simulink model "enable_test"  (Simulink 9.0)
settings: Solver=FixedStepDiscrete  StartTime=0.0  StopTime=1  FixedStep=1.000000  MaxStep=1  RelTol=1e-3  EnableMultiTasking=on
undefined symbols (not defined in the file): DiscIntNeverNeededParam
libraries: simulink x1
settings Model: SuppressorTable=22 serialization::archive 11 0 6 0 0 0 0 0  Creator=arnaud  LastModifiedBy=hbourbou
settings DataIOCC: ExternalInput=xin  LimitDataPoints=on  SaveFormat=StructureWithTime
settings DebuggingCC: UnderspecifiedInitializationDetection=Simplified  MergeDetectMultiDrivingBlocksExec=error  SolverPrmCheckMsg=warning
settings GRTTargetCC: GeneratePreprocessorConditionals=Disable all
settings ConfigComp: CovSFcnEnable=off

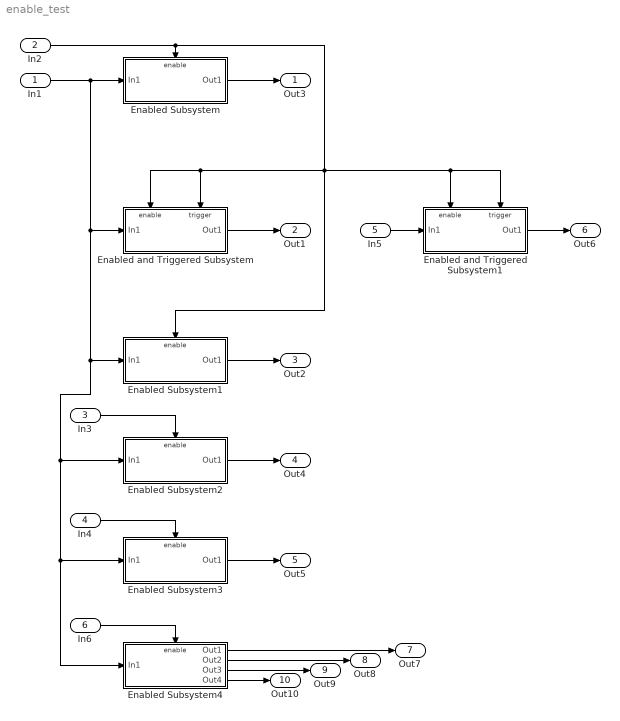
== system enable_test ==
  In1 : Inport
  In2 : Inport  Port=2  OutDataTypeStr=boolean
  In3 : Inport  Port=3  OutDataTypeStr=int8  PortDimensions=3
  In4 : Inport  Port=4  OutDataTypeStr=double
  In5 : Inport  Port=5
  In6 : Inport  Port=6  OutDataTypeStr=double
  Enabled Subsystem : Subsystem  TreatAsAtomicUnit=on
  Enabled Subsystem1 : Subsystem  TreatAsAtomicUnit=on
  Enabled Subsystem2 : Subsystem  TreatAsAtomicUnit=on
  Enabled Subsystem3 : Subsystem  TreatAsAtomicUnit=on
  Enabled Subsystem4 : Subsystem  TreatAsAtomicUnit=on
  Enabled and Triggered Subsystem : Subsystem  TreatAsAtomicUnit=on
  Enabled and Triggered Subsystem1 : Subsystem  TreatAsAtomicUnit=on
  Out3 : Outport
  Out1 : Outport  Port=2
  Out2 : Outport  Port=3
  Out4 : Outport  Port=4
  Out5 : Outport  Port=5
  Out6 : Outport  Port=6
  Out7 : Outport  Port=7
  Out8 : Outport  Port=8
  Out9 : Outport  Port=9
  Out10 : Outport  Port=10
  wires:
  Enabled Subsystem/1(Out1) -> Out3/1
  In2/1 -> Enabled and Triggered Subsystem1/Trigger, Enabled and Triggered Subsystem1/Enable, Enabled Subsystem1/Enable, Enabled and Triggered Subsystem/Trigger, Enabled and Triggered Subsystem/Enable, Enabled Subsystem/Enable
  Enabled and Triggered Subsystem/1(Out1) -> Out1/1
  Enabled Subsystem1/1(Out1) -> Out2/1
  Enabled Subsystem2/1(Out1) -> Out4/1
  Enabled Subsystem3/1(Out1) -> Out5/1
  In3/1 -> Enabled Subsystem2/Enable
  In4/1 -> Enabled Subsystem3/Enable
  Enabled and Triggered Subsystem1/1(Out1) -> Out6/1
  In5/1 -> Enabled and Triggered Subsystem1/1(In1)
  In1/1 -> Enabled Subsystem4/1(In1), Enabled Subsystem3/1(In1), Enabled Subsystem2/1(In1), Enabled Subsystem1/1(In1), Enabled and Triggered Subsystem/1(In1), Enabled Subsystem/1(In1)
  Enabled Subsystem4/1(Out1) -> Out7/1
  In6/1 -> Enabled Subsystem4/Enable
  Enabled Subsystem4/2(Out2) -> Out8/1
  Enabled Subsystem4/3(Out3) -> Out9/1
  Enabled Subsystem4/4(Out4) -> Out10/1

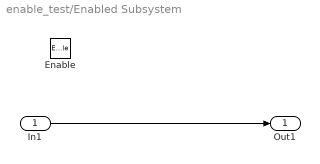
== system enable_test/Enabled Subsystem ==
  In1 : Inport
  Enable : EnablePort
  Out1 : Outport
  wires:
  In1/1 -> Out1/1

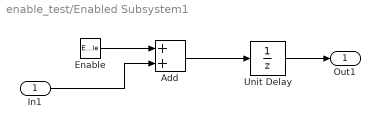
== system enable_test/Enabled Subsystem1 ==
  In1 : Inport
  Enable : EnablePort  StatesWhenEnabling=reset  ShowOutputPort=on
  Add : Sum
  Unit Delay : UnitDelay  SampleTime=-1
  Out1 : Outport
  wires:
  Enable/1 -> Add/1
  In1/1 -> Add/2
  Add/1 -> Unit Delay/1
  Unit Delay/1 -> Out1/1

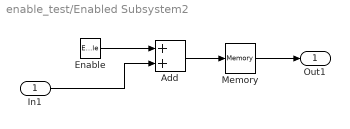
== system enable_test/Enabled Subsystem2 ==
  In1 : Inport
  Enable : EnablePort  StatesWhenEnabling=reset  ShowOutputPort=on
  Add : Sum
  Memory : Memory
  Out1 : Outport
  wires:
  Enable/1 -> Add/1
  In1/1 -> Add/2
  Add/1 -> Memory/1
  Memory/1 -> Out1/1

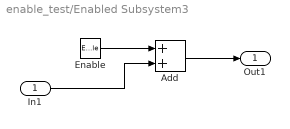
== system enable_test/Enabled Subsystem3 ==
  In1 : Inport
  Enable : EnablePort  ShowOutputPort=on
  Add : Sum
  Out1 : Outport
  wires:
  Enable/1 -> Add/1
  In1/1 -> Add/2
  Add/1 -> Out1/1

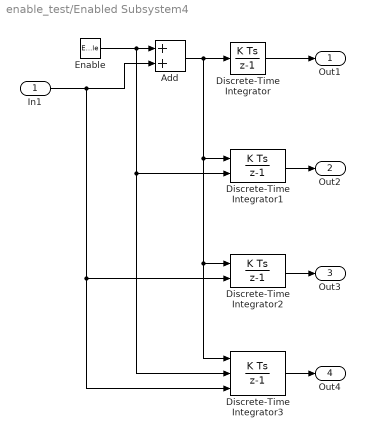
== system enable_test/Enabled Subsystem4 ==
  In1 : Inport
  Enable : EnablePort  StatesWhenEnabling=reset  ShowOutputPort=on
  Add : Sum
  Discrete-Time Integrator : DiscreteIntegrator  InitialConditionSetting=State (most efficient)  ICPrevOutput=DiscIntNeverNeededParam  ICPrevScaledInput=DiscIntNeverNeededParam
  Discrete-Time Integrator1 : DiscreteIntegrator  ExternalReset=falling  InitialConditionSetting=State (most efficient)  ICPrevOutput=DiscIntNeverNeededParam  ICPrevScaledInput=DiscIntNeverNeededParam
  Discrete-Time Integrator2 : DiscreteIntegrator  InitialConditionSource=external  InitialConditionSetting=State (most efficient)  ICPrevOutput=DiscIntNeverNeededParam  ICPrevScaledInput=DiscIntNeverNeededParam
  Discrete-Time Integrator3 : DiscreteIntegrator  ExternalReset=level  InitialConditionSource=external  InitialConditionSetting=State (most efficient)  ICPrevOutput=DiscIntNeverNeededParam  ICPrevScaledInput=DiscIntNeverNeededParam
  Out1 : Outport
  Out2 : Outport  Port=2
  Out3 : Outport  Port=3
  Out4 : Outport  Port=4
  wires:
  Enable/1 -> Discrete-Time Integrator3/2, Discrete-Time Integrator1/2, Add/1
  In1/1 -> Discrete-Time Integrator3/3, Discrete-Time Integrator2/2, Add/2
  Add/1 -> Discrete-Time Integrator3/1, Discrete-Time Integrator2/1, Discrete-Time Integrator1/1, Discrete-Time Integrator/1
  Discrete-Time Integrator/1 -> Out1/1
  Discrete-Time Integrator1/1 -> Out2/1
  Discrete-Time Integrator2/1 -> Out3/1
  Discrete-Time Integrator3/1 -> Out4/1

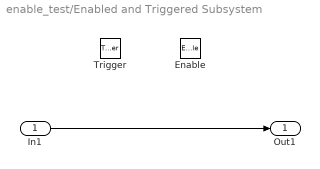
== system enable_test/Enabled and Triggered Subsystem ==
  In1 : Inport
  Enable : EnablePort
  Trigger : TriggerPort  VariantControl=(inherit)
  Out1 : Outport
  wires:
  In1/1 -> Out1/1

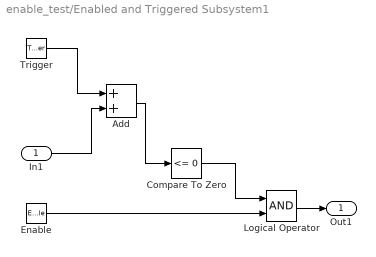
== system enable_test/Enabled and Triggered Subsystem1 ==
  In1 : Inport
  Enable : EnablePort  ShowOutputPort=on
  Trigger : TriggerPort  TriggerType=falling  VariantControl=(inherit)  ShowOutputPort=on
  Add : Sum
  Compare To Zero : simulink/Logic and Bit Operations/Compare To Zero  relop=<=  OutDataTypeStr=boolean
  Logical Operator : Logic  AllPortsSameDT=off  OutDataTypeStr=boolean
  Out1 : Outport
  wires:
  In1/1 -> Add/2
  Trigger/1 -> Add/1
  Add/1 -> Compare To Zero/1
  Enable/1 -> Logical Operator/2
  Logical Operator/1 -> Out1/1
  Compare To Zero/1 -> Logical Operator/1
